simulink model "monitor"  (R2021a)
settings: Solver=FixedStepAuto  StartTime=0.0  StopTime=10.0  RelTol=1e-3  EnableMultiTasking=on
settings Model: DataDictionary=worldDD.sldd  SILPILModeSetting=veronly  ExtModeTrigDuration=2  Creator=Koorosh  LastModifiedBy=Koorosh
settings OptimizationCC: EnhancedBackFolding=on  PassReuseOutputArgsAs=Individual arguments  ZeroExternalMemoryAtStartup=off  ZeroInternalMemoryAtStartup=off  MaxStackSize=64  OptimizeBlockOrder=speed  DifferentSizesBufferReuse=on  OptimizationCustomize=off  EfficientTunableParamExpr=on
settings DebuggingCC: ParameterTunabilityLossMsg=error
settings HardwareCC: ProdBitPerInt=16  ProdBitPerPointer=16  ProdBitPerSizeT=16  ProdBitPerPtrDiffT=16  ProdLargestAtomicFloat=None  ProdWordSize=8  ProdHWDeviceType=Atmel->AVR
settings SFSimCC: MATLABDynamicMemAlloc=off
settings RTWCC: SystemTargetFile=ert.tlc  HardwareBoard=Arduino Uno  TemplateMakefile=ert_default_tmf  Toolchain=Arduino AVR  BuildConfiguration=Faster Runs
settings CodeAppCC: ForceParamTrailComments=on  IgnoreCustomStorageClasses=off  OperatorAnnotations=on  SimulinkDataObjDesc=on  SFDataObjDesc=on  InsertBlockDesc=on
settings ERTTargetCC: SupportContinuousTime=on  SupportVariableSizeSignals=on  ExtModeStaticAllocSize=250

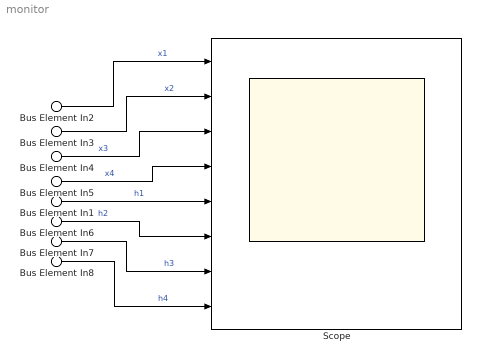
== system monitor ==
  Bus Element In2 : Inport  PortName=X  Element=x1
  Bus Element In3 : Inport  PortName=X  Element=x2
  Bus Element In4 : Inport  PortName=X  Element=x3
  Bus Element In5 : Inport  PortName=X  Element=x4
  Bus Element In1 : Inport  Port=2  PortName=H  Element=h1
  Bus Element In6 : Inport  Port=2  PortName=H  Element=h2
  Bus Element In7 : Inport  Port=2  PortName=H  Element=h3
  Bus Element In8 : Inport  Port=2  PortName=H  Element=h4
  Scope : Scope  NumInputPorts=8
  wires:
  Bus Element In2/1 -> Scope/1  "x1"
  Bus Element In3/1 -> Scope/2  "x2"
  Bus Element In4/1 -> Scope/3  "x3"
  Bus Element In5/1 -> Scope/4  "x4"
  Bus Element In1/1 -> Scope/5  "h1"
  Bus Element In6/1 -> Scope/6  "h2"
  Bus Element In7/1 -> Scope/7  "h3"
  Bus Element In8/1 -> Scope/8  "h4"
